simulink model "simulink_drone_sim_PID_all_open"  (R2025b)
settings: Solver=VariableStepAuto  StartTime=0.0  StopTime=10.0  RelTol=1e-3
settings Model: Creator=xuwan  LastModifiedBy=xuwan

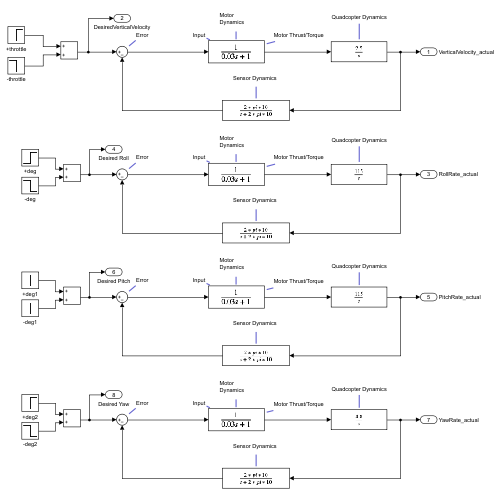
[thumbnail: Simulink's stored preview of the top-level diagram]
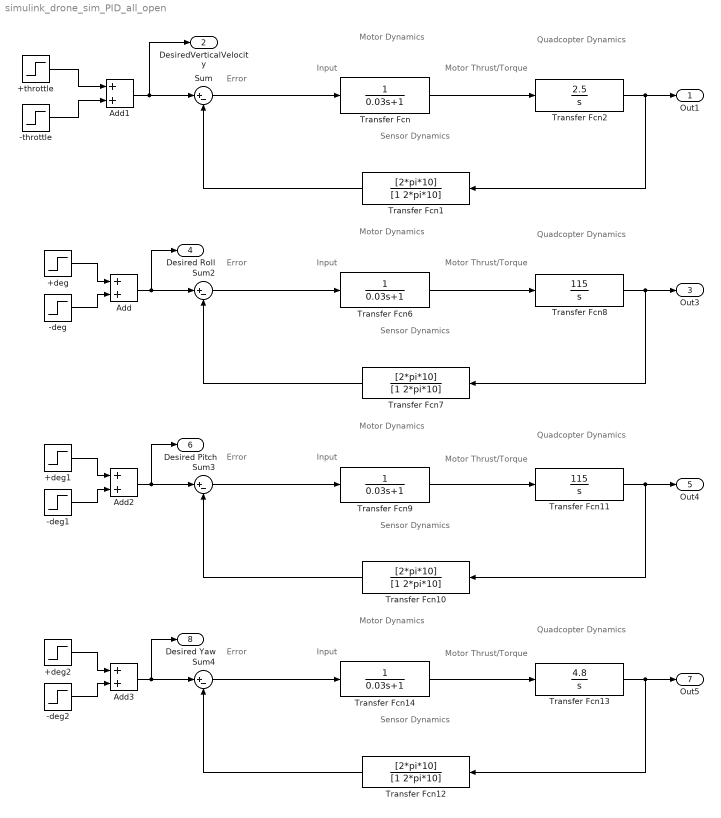
== system simulink_drone_sim_PID_all_open ==
  note: Motor Thrust/Torque
  note: Input
  note: Error
  note: Quadcopter Dynamics
  note: Sensor Dynamics
  note: Motor Dynamics
  note: Error
  note: Input
  note: Quadcopter Dynamics
  note: Motor Thrust/Torque
  note: Sensor Dynamics
  note: Motor Dynamics
  note: Sensor Dynamics
  note: Motor Dynamics
  note: Input
  note: Motor Thrust/Torque
  note: Error
  note: Quadcopter Dynamics
  note: Quadcopter Dynamics
  note: Motor Dynamics
  note: Input
  note: Error
  note: Sensor Dynamics
  note: Motor Thrust/Torque
  +deg : Step  Time=3  After=30  SampleTime=0
  +deg1 : Step  Time=3  After=30  SampleTime=0
  +deg2 : Step  Time=3  After=30  SampleTime=0
  +throttle : Step  After=10  SampleTime=0
  -deg : Step  Time=5  After=-30  SampleTime=0
  -deg1 : Step  Time=5  After=-30  SampleTime=0
  -deg2 : Step  Time=5  After=-30  SampleTime=0
  -throttle : Step  Time=5  After=-10  SampleTime=0
  Add{,1..3} (4 alike) : Sum
  Sum{,2..4} (4 alike) : Sum  Inputs=|+-
  Transfer Fcn{,6,9,14} (4 alike) : TransferFcn  Denominator=[0.03 1]
  Transfer Fcn{1,7,10,12} (4 alike) : TransferFcn  Numerator=[2*pi*10]  Denominator=[1 2*pi*10]
  Transfer Fcn11 : TransferFcn  Numerator=[115]  Denominator=[1 0]
  Transfer Fcn13 : TransferFcn  Numerator=[4.8]  Denominator=[1 0]
  Transfer Fcn2 : TransferFcn  Numerator=[2.5]  Denominator=[1 0]
  Transfer Fcn8 : TransferFcn  Numerator=[115]  Denominator=[1 0]
  Out1 : Outport  SignalName=VerticalVelocity_actual
  DesiredVerticalVelocity : Outport  Port=2
  Out3 : Outport  Port=3  SignalName=RollRate_actual
  Desired Roll : Outport  Port=4
  Out4 : Outport  Port=5  SignalName=PitchRate_actual
  Desired Pitch : Outport  Port=6
  Out5 : Outport  Port=7  SignalName=YawRate_actual
  Desired Yaw : Outport  Port=8
  wires:
  Transfer Fcn/1 -> Transfer Fcn2/1
  Transfer Fcn2/1 -> Out1/1, Transfer Fcn1/1
  Transfer Fcn1/1 -> Sum/2
  Sum/1 -> Transfer Fcn/1
  Transfer Fcn6/1 -> Transfer Fcn8/1
  Transfer Fcn7/1 -> Sum2/2
  Sum2/1 -> Transfer Fcn6/1
  +deg/1 -> Add/1
  -deg/1 -> Add/2
  Transfer Fcn8/1 -> Out3/1, Transfer Fcn7/1
  Add/1 -> Desired Roll/1, Sum2/1
  Add1/1 -> DesiredVerticalVelocity/1, Sum/1
  +throttle/1 -> Add1/1
  -throttle/1 -> Add1/2
  +deg1/1 -> Add2/1
  Sum3/1 -> Transfer Fcn9/1
  Transfer Fcn9/1 -> Transfer Fcn11/1
  Add2/1 -> Desired Pitch/1, Sum3/1
  Transfer Fcn10/1 -> Sum3/2
  -deg1/1 -> Add2/2
  Transfer Fcn11/1 -> Out4/1, Transfer Fcn10/1
  Transfer Fcn14/1 -> Transfer Fcn13/1
  Sum4/1 -> Transfer Fcn14/1
  Transfer Fcn12/1 -> Sum4/2
  +deg2/1 -> Add3/1
  Add3/1 -> Desired Yaw/1, Sum4/1
  -deg2/1 -> Add3/2
  Transfer Fcn13/1 -> Out5/1, Transfer Fcn12/1
